simulink model "project_rectifier_withbuck"  (R2025a)
settings: Solver=VariableStepAuto  StartTime=0.0  StopTime=4  RelTol=1e-3
libraries: spsSeriesRLCBranchLib x6, spsVoltageMeasurementLib x6, spsDiodeLib x5, spsCurrentMeasurementLib x4, spsACVoltageSourceLib x1, spsDCMachineLib x1, spsDCVoltageSourceLib x1, spsMosfetLib x1, spsNeutralLib x1, spsPWMGeneratorDCDCLib x1, sps_lib x1
settings Model: Creator=em  LastModifiedBy=em
settings SolverCC: ZeroCrossAlgorithm=Adaptive

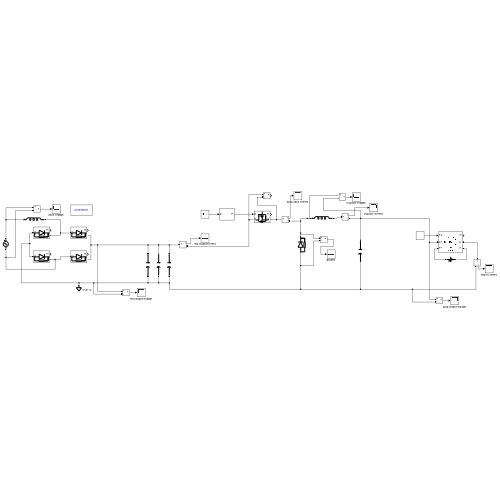
[thumbnail: Simulink's stored preview of the top-level diagram]
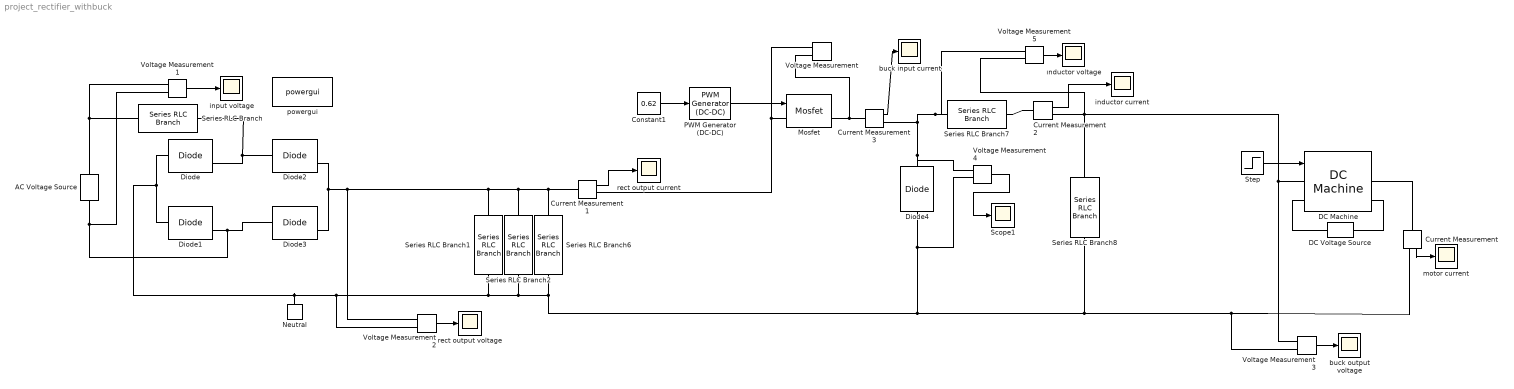
== system project_rectifier_withbuck ==
  AC Voltage Source : spsACVoltageSourceLib/AC Voltage Source  Amplitude=230*sqrt(2)  Phase=0  Frequency=50  SampleTime=2e-6  Measurements=None  BusType=swing  Pref=10e3  Qref=0  Qmin=-inf  Qmax=+inf
  Constant1 : Constant  Value=0.62
  Current Measurement{,1..3} (4 alike) : spsCurrentMeasurementLib/Current Measurement  PhasorSimulation=off  OutputType=Complex  PSBequivalent=0
  DC Machine : spsDCMachineLib/DC Machine  PresetModel=No  MechanicalLoad=Torque TL  FieldType=Wound  ShowDetailedParameters=on  MeasurementBus=off  RLa=[0.6 0.012]  RLf=[220 120]  Laf=1.31  MachineConstant=Torque constant (N.m/A)  Ke=1.8  Kt=1.8  J=0.05  Bm=0.008  Tf=0.5  w0=0  Ifinit=0.999999998825435  TsPowergui=0  TsBlock=-1
  DC Voltage Source : spsDCVoltageSourceLib/DC Voltage Source  Amplitude=220  Measurements=None
  Diode{,1..3} (4 alike) : spsDiodeLib/Diode  Ron=0.001  Lon=0  Vf=0.6  IC=0  UseSnubber=0  Rs=500  Cs=250e-9  Measurements=on
  Diode4 : spsDiodeLib/Diode  Ron=0.001  Lon=0  Vf=0.8  IC=0  UseSnubber=0  Rs=500  Cs=250e-9  Measurements=off
  Mosfet : spsMosfetLib/Mosfet  Ron=0.1  Lon=0  Rd=0.01  Vfd=0  IC=0  Rs=1e5  Cs=inf  Measurements=on
  Neutral : spsNeutralLib/Neutral  LConnTagsString=a  NodeNumber=10
      settings: AttributesFormatString=node %<NodeNumber>  LibrarySourceBlock=sps_lib/Utilities/Neutral
  PWM Generator (DC-DC) : spsPWMGeneratorDCDCLib/PWM Generator (DC-DC)  Fsw=30000  Ts=0
  Scope1 : Scope
      settings: DataLoggingVariableName=ScopeData7
  Series RLC Branch : spsSeriesRLCBranchLib/Series RLC Branch  LConnTagsString=__new0  RConnTagsString=__new0  BranchType=L  Resistance=1  Inductance=2e-3  SetiL0=off  InitialCurrent=0  Capacitance=1e-6  Setx0=off  InitialVoltage=0  Measurements=None
  Series RLC Branch1 : spsSeriesRLCBranchLib/Series RLC Branch  LConnTagsString=__new0  RConnTagsString=__new0  BranchType=C  Resistance=1  Inductance=1e-3  SetiL0=off  InitialCurrent=0  Capacitance=470e-6  Setx0=off  InitialVoltage=0  Measurements=None
  Series RLC Branch2 : spsSeriesRLCBranchLib/Series RLC Branch  LConnTagsString=__new0  RConnTagsString=__new0  BranchType=C  Resistance=1  Inductance=1e-3  SetiL0=off  InitialCurrent=0  Capacitance=470e-6  Setx0=off  InitialVoltage=0  Measurements=None
  Series RLC Branch6 : spsSeriesRLCBranchLib/Series RLC Branch  LConnTagsString=__new0  RConnTagsString=__new0  BranchType=C  Resistance=1  Inductance=1e-3  SetiL0=off  InitialCurrent=0  Capacitance=10e-9  Setx0=off  InitialVoltage=0  Measurements=None
  Series RLC Branch7 : spsSeriesRLCBranchLib/Series RLC Branch  LConnTagsString=__new0  RConnTagsString=__new0  BranchType=L  Resistance=1  Inductance=1e-3  SetiL0=off  InitialCurrent=0  Capacitance=1e-6  Setx0=off  InitialVoltage=0  Measurements=None
  Series RLC Branch8 : spsSeriesRLCBranchLib/Series RLC Branch  LConnTagsString=__new0  RConnTagsString=__new0  BranchType=C  Resistance=0.025  Inductance=1e-3  SetiL0=off  InitialCurrent=0  Capacitance=470e-6  Setx0=off  InitialVoltage=0  Measurements=None
  Step : Step  Time=0  After=15  SampleTime=0
  Voltage Measurement{,1..5} (6 alike) : spsVoltageMeasurementLib/Voltage Measurement  PhasorSimulation=off  OutputType=Complex  PSBequivalent=0
  buck input current : Scope
      settings: ActiveDisplayYMinimum=-1.1034224934030235  ActiveDisplayYMaximum=21.407344193774449  DataLoggingVariableName=ScopeData6
  buck output voltage : Scope
      settings: ActiveDisplayYMinimum=160.32586557215177  ActiveDisplayYMaximum=241.23455220664673
  inductor current : Scope
      settings: ActiveDisplayYMinimum=-6.1614939490169558  ActiveDisplayYMaximum=54.896698004916828  DataLoggingVariableName=ScopeData5
  input voltage : Scope
      settings: ActiveDisplayYMinimum=-363.52795393811232  ActiveDisplayYMaximum=342.51616176058508
  motor current : Scope
      settings: ActiveDisplayYMinimum=-34.6108275231653  ActiveDisplayYMaximum=283.34634117406119  DataLoggingVariableName=ScopeData2
  powergui : sps_lib/powergui  Priority=1  SimulationMode=Continuous  SampleTime=50e-6  frequency=50  Iterations=50  frequencyindice=50  Pbase=100e6  ErrMax=1e-4  UnitsV=kV  UnitsW=MW  buscounter=0  FunctionMessages=off  echomessages=off  EnableUseOfTLC=off  CurrentSourceSwitches=off  DisableSnubberDevices=off  DisableRonSwitches=off  DisableVfSwitches=off  DisplayEquations=off  AutomaticDiscreteSolvers=off  SolverType=Tustin/Backward Euler (TBE)  Interpol=off  ExternalGateDelay=off  methode=off  Ts=100  x0status=blocks  SPID=on  SwTol=0  HookPort=off  NonlinearTolerance=1e-4  nMaxIteration=100  ContinueOnMaxIteration=off  RestoreLinks=warning  ResistiveCurrentMeasurement=off  Frange=[0:2:500]  Ylog=off  Xlog=on  ShowGrid=off  save=off  variable=ZData  structure=0  ZoomFFT=off  StartTime=0.0  cycles=1  DisplayStyle=1  fundamental=60  FreqAxis=off  MaxFrequency=1000  frequencyindicesteady=1  RmsSteady=1  display=off
  rect output current : Scope
      settings: ActiveDisplayYMinimum=-34.6108275231653  ActiveDisplayYMaximum=283.34634117406119  DataLoggingVariableName=ScopeData4
  rect output voltage : Scope
      settings: ActiveDisplayYMinimum=-56.744245519825391  ActiveDisplayYMaximum=510.69820967842793  DataLoggingVariableName=ScopeData3
  ınductor voltage : Scope
      settings: ActiveDisplayYMinimum=-455.27902308986552  ActiveDisplayYMaximum=314.9001355052489  DataLoggingVariableName=ScopeData8
  wires:
  Voltage Measurement1/1 -> input voltage/1
  Current Measurement/1 -> motor current/1
  Voltage Measurement2/1 -> rect output voltage/1
  Voltage Measurement3/1 -> buck output voltage/1
  Current Measurement1/1 -> rect output current/1
  Constant1/1 -> PWM Generator (DC-DC)/1
  PWM Generator (DC-DC)/1 -> Mosfet/1
  Current Measurement3/1 -> buck input current/1
  Voltage Measurement4/1 -> Scope1/1
  Voltage Measurement5/1 -> ınductor voltage/1
  Current Measurement2/1 -> inductor current/1
  Step/1 -> DC Machine/1
  connections:
  Diode/RConn1 -- Series RLC Branch/RConn1 -- Diode2/LConn1
  Diode3/LConn1 -- Voltage Measurement1/LConn2 -- AC Voltage Source/LConn1 -- Diode1/RConn1
  Diode1/LConn1 -- Series RLC Branch8/RConn1 -- Current Measurement/RConn1 -- Voltage Measurement3/LConn2 -- Voltage Measurement4/LConn2 -- Diode4/LConn1 -- Series RLC Branch6/RConn1 -- Series RLC Branch2/RConn1 -- Series RLC Branch1/RConn1 -- Voltage Measurement2/LConn2 -- Neutral/LConn1 -- Diode/LConn1
  AC Voltage Source/RConn1 -- Voltage Measurement1/LConn1 -- Series RLC Branch/LConn1
  DC Machine/LConn2 -- DC Voltage Source/RConn1
  DC Voltage Source/LConn1 -- DC Machine/RConn2
  DC Machine/RConn1 -- Current Measurement/LConn1
  Series RLC Branch1/LConn1 -- Series RLC Branch6/LConn1 -- Current Measurement1/LConn1 -- Series RLC Branch2/LConn1 -- Voltage Measurement2/LConn1 -- Diode2/RConn1 -- Diode3/RConn1
  Mosfet/LConn1 -- Current Measurement1/RConn1 -- Voltage Measurement/LConn1
  Mosfet/RConn1 -- Current Measurement3/LConn1 -- Voltage Measurement/LConn2
  Diode4/RConn1 -- Voltage Measurement5/LConn1 -- Series RLC Branch7/LConn1 -- Current Measurement3/RConn1 -- Voltage Measurement4/LConn1
  DC Machine/LConn1 -- Voltage Measurement3/LConn1 -- Voltage Measurement5/LConn2 -- Series RLC Branch8/LConn1 -- Current Measurement2/RConn1
  Current Measurement2/LConn1 -- Series RLC Branch7/RConn1
